simulink model "Filter"  (R2020b)
settings: Solver=VariableStepAuto  StartTime=0.0  StopTime=10.0  RelTol=1e-3
libraries: dspvision x1
settings Model: Creator=ncleju  LastModifiedBy=ncleju

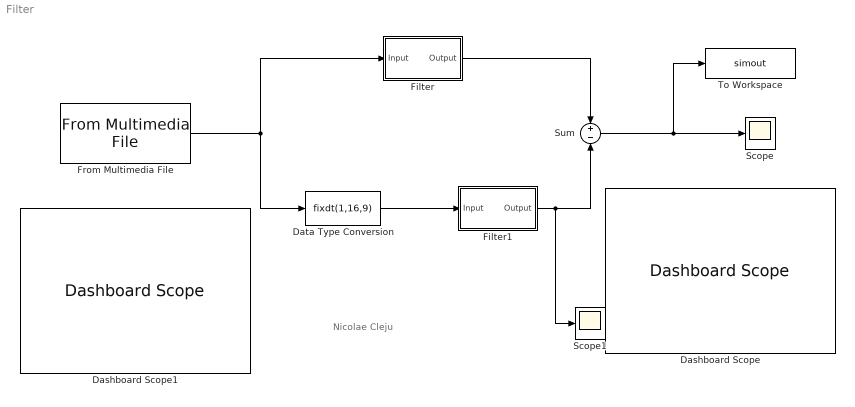
== system Filter ==
  note: Nicolae Cleju
  Dashboard Scope : DashboardScope
  Dashboard Scope1 : DashboardScope
  Data Type Conversion : DataTypeConversion  OutDataTypeStr=fixdt(1,16,9)
  Filter : Subsystem  Tag=FilterWizardSubSystem
      settings: ErrorFcn=dspFilterRealizedInBasicElemsAlgLoopErrFcnCallback
  Filter1 : Subsystem  Tag=FilterWizardSubSystem
      settings: ErrorFcn=dspFilterRealizedInBasicElemsAlgLoopErrFcnCallback
  From Multimedia File : dspvision/From Multimedia File  inputFilename=speech_dft.mp3  readRange=[1 Inf]  loop=on  numPlays=inf  outputStreams=Audio only  videoDataType=single  audioDataType=double  inheritSampleTime=on  userDefinedSampleTime=1/30  noAudioOutput=off  isIntensityVideo=off  fourcc=RGB  colorVideoFormat=Separate color signals  outputEOF=off  dataOrg=Column-major  audioFrameSize=1  computeAudioFrameSize=off  outSamplingMode=Sample based
  Scope : Scope
  Scope1 : Scope
  Sum : Sum  Inputs=+|-
  To Workspace : ToWorkspace  VariableName=simout  SampleTime=-1
  wires:
  From Multimedia File/1 -> Filter/1(Input), Data Type Conversion/1
  Filter/1(Output) -> Sum/1
  Filter1/1(Output) -> Scope1/1, Sum/2
  Sum/1 -> To Workspace/1, Scope/1
  Data Type Conversion/1 -> Filter1/1(Input)

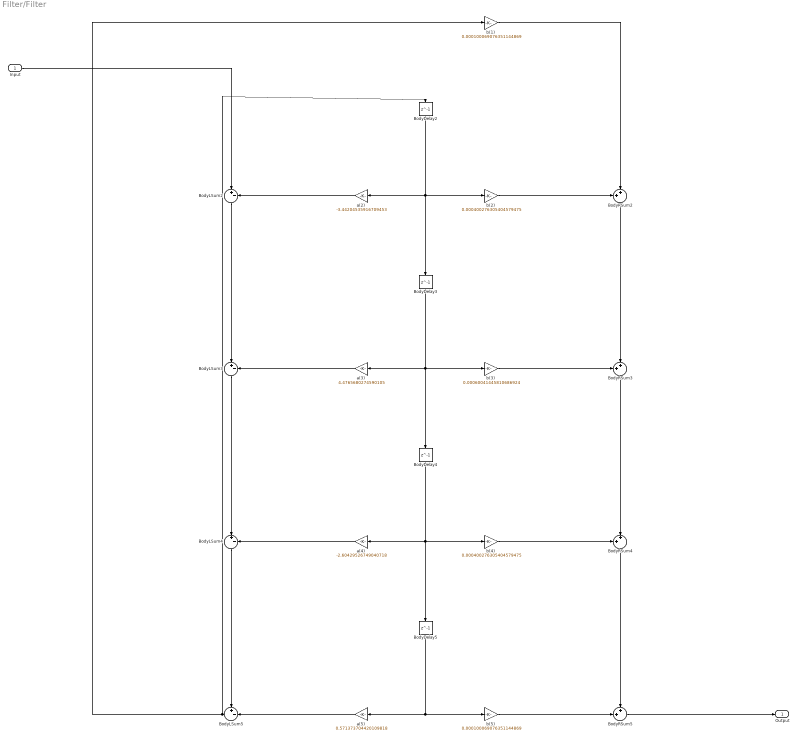
== system Filter/Filter ==
  Input : Inport
  BodyDelay{2..5} (4 alike) : Delay  DelayLength=1  InitialCondition=0
  BodyLSum2 : Sum  Inputs=|+-  RndMeth=Nearest  SaturateOnIntegerOverflow=on  OutDataTypeStr=Inherit: Same as first input
  BodyLSum3 : Sum  Inputs=|+-  RndMeth=Nearest  SaturateOnIntegerOverflow=on  OutDataTypeStr=Inherit: Same as first input
  BodyLSum4 : Sum  Inputs=|+-  RndMeth=Nearest  SaturateOnIntegerOverflow=on  OutDataTypeStr=Inherit: Same as first input
  BodyLSum5 : Sum  Inputs=+-|  RndMeth=Nearest  SaturateOnIntegerOverflow=on  OutDataTypeStr=Inherit: Same as first input
  BodyRSum{2..5} (4 alike) : Sum  Inputs=++|  RndMeth=Nearest  SaturateOnIntegerOverflow=on  OutDataTypeStr=Inherit: Same as first input
  a(2) : Gain  Gain=-3.44204535916709453  ParamDataTypeStr=double  RndMeth=Nearest  SaturateOnIntegerOverflow=on  OutDataTypeStr=Inherit: Same as input
  a(3) : Gain  Gain=4.4765680274590105  ParamDataTypeStr=double  RndMeth=Nearest  SaturateOnIntegerOverflow=on  OutDataTypeStr=Inherit: Same as input
  a(4) : Gain  Gain=-2.60429526749040718  ParamDataTypeStr=double  RndMeth=Nearest  SaturateOnIntegerOverflow=on  OutDataTypeStr=Inherit: Same as input
  a(5) : Gain  Gain=0.571373704420109818  ParamDataTypeStr=double  RndMeth=Nearest  SaturateOnIntegerOverflow=on  OutDataTypeStr=Inherit: Same as input
  b(1) : Gain  Gain=0.000100069076351144869  ParamDataTypeStr=double  RndMeth=Nearest  SaturateOnIntegerOverflow=on  OutDataTypeStr=Inherit: Same as input
  b(2) : Gain  Gain=0.000400276305404579475  ParamDataTypeStr=double  RndMeth=Nearest  SaturateOnIntegerOverflow=on  OutDataTypeStr=Inherit: Same as input
  b(3) : Gain  Gain=0.00060041445810686924  ParamDataTypeStr=double  RndMeth=Nearest  SaturateOnIntegerOverflow=on  OutDataTypeStr=Inherit: Same as input
  b(4) : Gain  Gain=0.000400276305404579475  ParamDataTypeStr=double  RndMeth=Nearest  SaturateOnIntegerOverflow=on  OutDataTypeStr=Inherit: Same as input
  b(5) : Gain  Gain=0.000100069076351144869  ParamDataTypeStr=double  RndMeth=Nearest  SaturateOnIntegerOverflow=on  OutDataTypeStr=Inherit: Same as input
  Output : Outport
  wires:
  b(1)/1 -> BodyRSum2/2
  Input/1 -> BodyLSum2/1
  BodyLSum2/1 -> BodyLSum3/1
  a(2)/1 -> BodyLSum2/2
  BodyDelay2/1 -> a(2)/1, b(2)/1, BodyDelay3/1
  b(2)/1 -> BodyRSum2/1
  BodyRSum2/1 -> BodyRSum3/2
  BodyLSum3/1 -> BodyLSum4/1
  a(3)/1 -> BodyLSum3/2
  BodyDelay3/1 -> a(3)/1, b(3)/1, BodyDelay4/1
  b(3)/1 -> BodyRSum3/1
  BodyRSum3/1 -> BodyRSum4/2
  BodyLSum4/1 -> BodyLSum5/1
  a(4)/1 -> BodyLSum4/2
  BodyDelay4/1 -> a(4)/1, b(4)/1, BodyDelay5/1
  b(4)/1 -> BodyRSum4/1
  BodyRSum4/1 -> BodyRSum5/1
  BodyLSum5/1 -> b(1)/1, BodyDelay2/1
  a(5)/1 -> BodyLSum5/2
  BodyDelay5/1 -> a(5)/1, b(5)/1
  b(5)/1 -> BodyRSum5/2
  BodyRSum5/1 -> Output/1

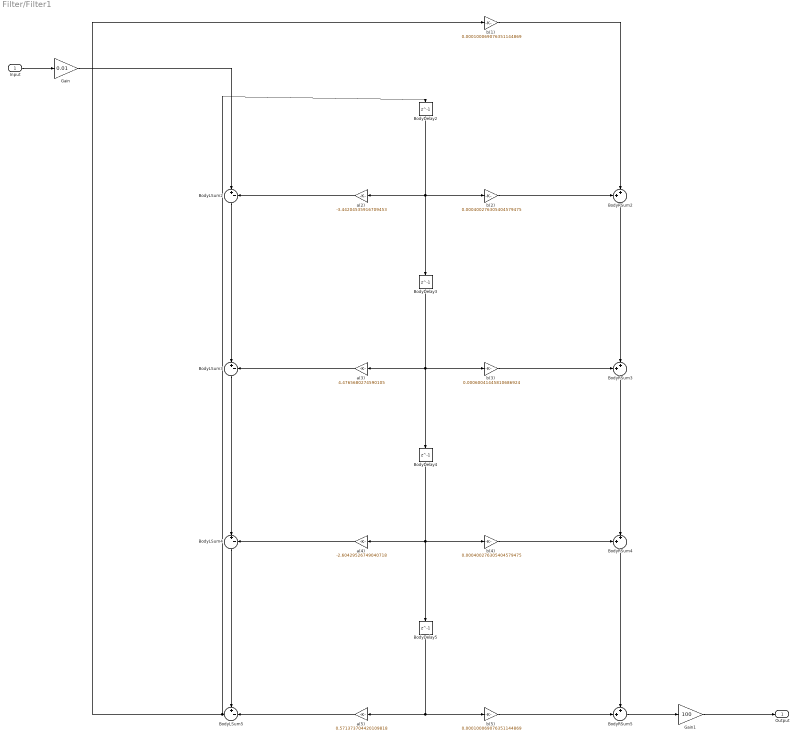
== system Filter/Filter1 ==
  Input : Inport
  BodyDelay{2..5} (4 alike) : Delay  DelayLength=1  InitialCondition=0
  BodyLSum2 : Sum  Inputs=|+-  RndMeth=Nearest  SaturateOnIntegerOverflow=on  OutDataTypeStr=Inherit: Same as first input
  BodyLSum3 : Sum  Inputs=|+-  RndMeth=Nearest  SaturateOnIntegerOverflow=on  OutDataTypeStr=Inherit: Same as first input
  BodyLSum4 : Sum  Inputs=|+-  RndMeth=Nearest  SaturateOnIntegerOverflow=on  OutDataTypeStr=Inherit: Same as first input
  BodyLSum5 : Sum  Inputs=+-|  RndMeth=Nearest  SaturateOnIntegerOverflow=on  OutDataTypeStr=Inherit: Same as first input
  BodyRSum{2..5} (4 alike) : Sum  Inputs=++|  RndMeth=Nearest  SaturateOnIntegerOverflow=on  OutDataTypeStr=Inherit: Same as first input
  Gain : Gain  Gain=0.01  OutDataTypeStr=Inherit: Same as input
  Gain1 : Gain  Gain=100  OutDataTypeStr=Inherit: Same as input
  a(2) : Gain  Gain=-3.44204535916709453  ParamDataTypeStr=double  RndMeth=Nearest  SaturateOnIntegerOverflow=on  OutDataTypeStr=Inherit: Same as input
  a(3) : Gain  Gain=4.4765680274590105  ParamDataTypeStr=double  RndMeth=Nearest  SaturateOnIntegerOverflow=on  OutDataTypeStr=Inherit: Same as input
  a(4) : Gain  Gain=-2.60429526749040718  ParamDataTypeStr=double  RndMeth=Nearest  SaturateOnIntegerOverflow=on  OutDataTypeStr=Inherit: Same as input
  a(5) : Gain  Gain=0.571373704420109818  ParamDataTypeStr=double  RndMeth=Nearest  SaturateOnIntegerOverflow=on  OutDataTypeStr=Inherit: Same as input
  b(1) : Gain  Gain=0.000100069076351144869  ParamDataTypeStr=double  RndMeth=Nearest  SaturateOnIntegerOverflow=on  OutDataTypeStr=Inherit: Same as input
  b(2) : Gain  Gain=0.000400276305404579475  ParamDataTypeStr=double  RndMeth=Nearest  SaturateOnIntegerOverflow=on  OutDataTypeStr=Inherit: Same as input
  b(3) : Gain  Gain=0.00060041445810686924  ParamDataTypeStr=double  RndMeth=Nearest  SaturateOnIntegerOverflow=on  OutDataTypeStr=Inherit: Same as input
  b(4) : Gain  Gain=0.000400276305404579475  ParamDataTypeStr=double  RndMeth=Nearest  SaturateOnIntegerOverflow=on  OutDataTypeStr=Inherit: Same as input
  b(5) : Gain  Gain=0.000100069076351144869  ParamDataTypeStr=double  RndMeth=Nearest  SaturateOnIntegerOverflow=on  OutDataTypeStr=Inherit: Same as input
  Output : Outport
  wires:
  b(1)/1 -> BodyRSum2/2
  Input/1 -> Gain/1
  BodyLSum2/1 -> BodyLSum3/1
  a(2)/1 -> BodyLSum2/2
  BodyDelay2/1 -> a(2)/1, b(2)/1, BodyDelay3/1
  b(2)/1 -> BodyRSum2/1
  BodyRSum2/1 -> BodyRSum3/2
  BodyLSum3/1 -> BodyLSum4/1
  a(3)/1 -> BodyLSum3/2
  BodyDelay3/1 -> a(3)/1, b(3)/1, BodyDelay4/1
  b(3)/1 -> BodyRSum3/1
  BodyRSum3/1 -> BodyRSum4/2
  BodyLSum4/1 -> BodyLSum5/1
  a(4)/1 -> BodyLSum4/2
  BodyDelay4/1 -> a(4)/1, b(4)/1, BodyDelay5/1
  b(4)/1 -> BodyRSum4/1
  BodyRSum4/1 -> BodyRSum5/1
  BodyLSum5/1 -> b(1)/1, BodyDelay2/1
  a(5)/1 -> BodyLSum5/2
  BodyDelay5/1 -> a(5)/1, b(5)/1
  b(5)/1 -> BodyRSum5/2
  BodyRSum5/1 -> Gain1/1
  Gain/1 -> BodyLSum2/1
  Gain1/1 -> Output/1
